simulink model "SingleJoint_PID"  (R2015b)
settings: Solver=VariableStepAuto  StartTime=0.0  StopTime=100  RelTol=1e-3
settings Model: Creator=wfxu  LastModifiedBy=wfxu

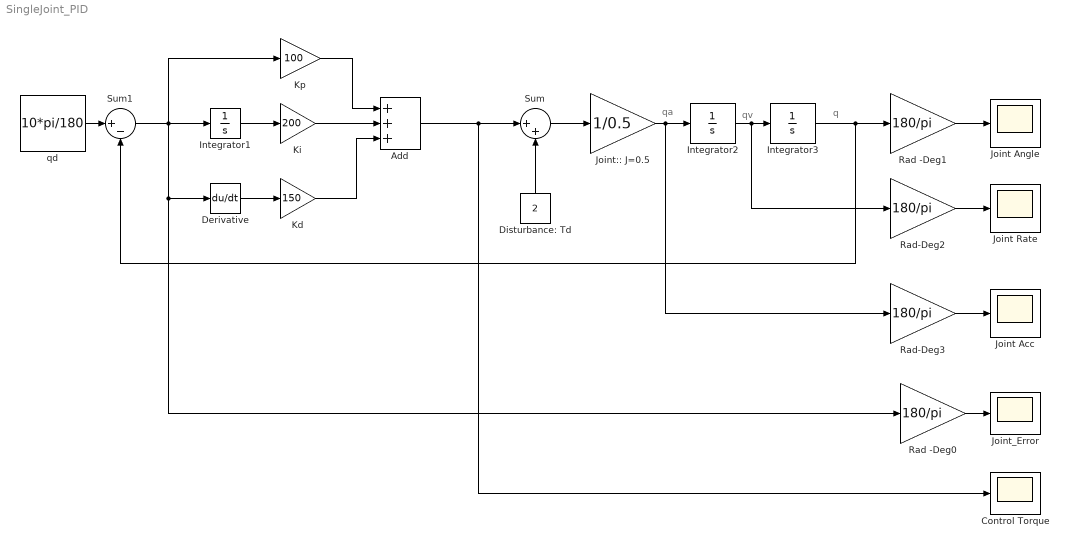
== system SingleJoint_PID ==
  note: qa
  note: qv
  note: q
  Add : Sum  Inputs=+++
  Control Torque : Scope
  Derivative : Derivative
  Disturbance: Td : Constant  Value=2
  Integrator1 : Integrator
  Integrator2 : Integrator
  Integrator3 : Integrator
  Joint Acc : Scope
  Joint Angle : Scope
  Joint Rate : Scope
  Joint:: J=0.5 : Gain  Gain=1/0.5
  Joint_Error : Scope
  Kd : Gain  Gain=150
  Ki : Gain  Gain=200
  Kp : Gain  Gain=100
  Rad -Deg0 : Gain  Gain=180/pi
  Rad -Deg1 : Gain  Gain=180/pi
  Rad-Deg2 : Gain  Gain=180/pi
  Rad-Deg3 : Gain  Gain=180/pi
  Sum : Sum  Inputs=|++
  Sum1 : Sum  Inputs=|+-
  qd : Constant  Value=10*pi/180
  wires:
  Integrator2/1 -> Rad-Deg2/1, Integrator3/1
  Joint:: J=0.5/1 -> Rad-Deg3/1, Integrator2/1
  Integrator3/1 -> Sum1/2, Rad -Deg1/1
  qd/1 -> Sum1/1
  Sum1/1 -> Rad -Deg0/1, Derivative/1, Kp/1, Integrator1/1
  Kp/1 -> Add/1
  Integrator1/1 -> Ki/1
  Ki/1 -> Add/2
  Derivative/1 -> Kd/1
  Kd/1 -> Add/3
  Rad -Deg1/1 -> Joint Angle/1
  Rad-Deg2/1 -> Joint Rate/1
  Rad-Deg3/1 -> Joint Acc/1
  Rad -Deg0/1 -> Joint_Error/1
  Add/1 -> Sum/1, Control Torque/1
  Disturbance: Td/1 -> Sum/2
  Sum/1 -> Joint:: J=0.5/1
